simulink model "demo_ADC_UDP"  (R2024b)
settings: Solver=VariableStepAuto  StartTime=0.0  StopTime=2  RelTol=1e-3
InitFcn:
  | Fs=5e3
  | Inter_sampling=0.5
libraries: dspnetwork x1
settings Model: PacingRate=4  Creator=77296  LastModifiedBy=77296

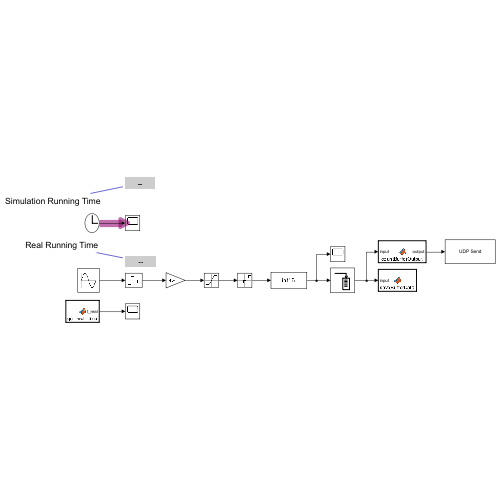
[thumbnail: Simulink's stored preview of the top-level diagram]
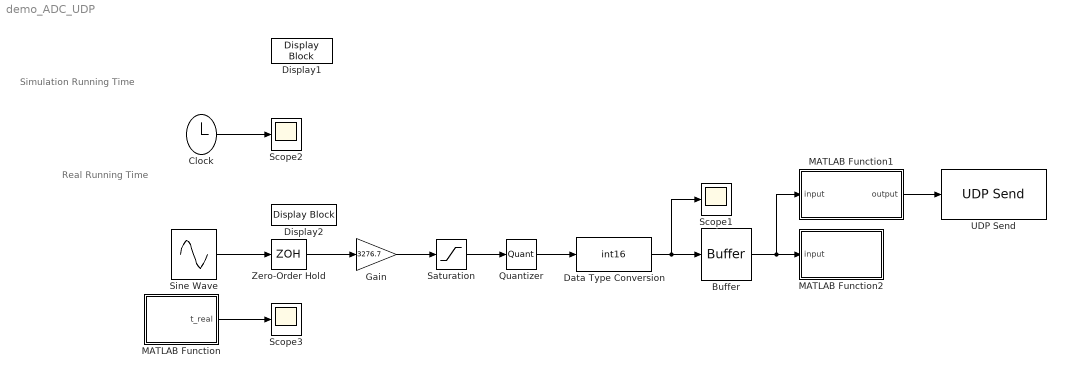
== system demo_ADC_UDP ==
  note: Real Running Time
  note: Simulation Running Time
  Buffer : Buffer  N=Fs*Inter_sampling  OutputFrames=off
  Clock : Clock
  Data Type Conversion : DataTypeConversion  OutMin=[-32768]  OutMax=[32767]  OutDataTypeStr=int16  RndMeth=Nearest  LockScale=on
  Display1 : DisplayBlock  LabelPosition=Hide  Transparency=1
  Display2 : DisplayBlock  LabelPosition=Hide  Transparency=1
  Gain : Gain  Gain=3276.7
  MATLAB Function : MATLAB Function  TreatAsAtomicUnit=on
  MATLAB Function1 : MATLAB Function  TreatAsAtomicUnit=on
  MATLAB Function2 : MATLAB Function  TreatAsAtomicUnit=on
  Quantizer : Quantizer  QuantizationInterval=20/65536
  Saturation : Saturate  UpperLimit=32767  LowerLimit=-32768
  Scope1 : Scope
  Scope2 : Scope
  Scope3 : Scope
  Sine Wave : Sin  Amplitude=10  Frequency=2*pi*50  SampleTime=0
  UDP Send : dspnetwork/UDP Send  remoteURL='110.110.110.108'  remotePort=5005  localURL='0.0.0.0'  localPortSource=Automatically determine  localPort=-1  sendBufferSize=Fs*Inter_sampling*2  sampletime=-1  blockPlatform=[]  separateLengthPort=0
      settings: LibrarySourceBlock=dspsnks4/UDP Send
  Zero-Order Hold : ZeroOrderHold  SampleTime=1/(Fs)
  wires:
  Quantizer/1 -> Data Type Conversion/1
  Buffer/1 -> MATLAB Function2/1(input), MATLAB Function1/1(input)
  Clock/1 -> Scope2/1
  Saturation/1 -> Quantizer/1
  Zero-Order Hold/1 -> Gain/1
  Sine Wave/1 -> Zero-Order Hold/1
  Gain/1 -> Saturation/1
  MATLAB Function/1(t_real) -> Scope3/1
  Data Type Conversion/1 -> Scope1/1, Buffer/1
  MATLAB Function1/1(output) -> UDP Send/1

== matlab function demo_ADC_UDP/MATLAB Function ==
  data: t_real output
function t_real = get_wall_time()
%#codegen
persistent t0
if isempty(t0)
    t0 = tic; % 记录仿真启动的实际时间
end
t_real = toc(t0); % 输出实际运行时间（秒）
end

== matlab function demo_ADC_UDP/MATLAB Function2 ==
  data: input input
function saveBufferData(input)
    persistent count;
    if isempty(count)
        count = int32(1);  % 初始化计数器并将其类型设置为 int32
    end

    % 使用 sprintf 动态生成变量名
    varName = sprintf('bufferData%d', count);  % 生成如 bufferData1, bufferData2 等变量名

    % 将数据保存到 Workspace
    assignin('base', varName, input);  % 将数据存储到基础 Workspace

    % 每次接收数据时增加计数
    count = count + 1;
end

== matlab function demo_ADC_UDP/MATLAB Function1 ==
  data: input input; output output
function output = countBufferOutput(input)
    persistent count;
    if isempty(count)
        count = 0;
    end
    count = count + 1;  % 每次收到输入时增加计数
    output = input;  % 保持输入数据不变
    
    % 强制转换 count 为 int32 类型，并显示输出次数
    disp('Output count:');  % 输出次数
    disp(count);  % 输出次数
    % 显示当前输入数据帧的长度
    frame_length = length(input);  % 获取当前帧的长度
    disp(sprintf('Frame length: %d', frame_length));  % 显示单个帧的长度
end
